simulink model "SMC_sim"  (R2024b)
settings: Solver=ode5  StartTime=0.0  StopTime=tf  FixedStep=dt  RelTol=1e-3
values from neighbouring files (symbols this model uses):
  A = double(subs(jacobian(x_dot, x_vars), [x_vars;u], [x_star; u_star]))    [inverted_pend_SMC.m]
  B = double(subs(jacobian(x_dot, u), [x_vars;u], [x_star; u_star]))    [inverted_pend_SMC.m]
  C = [1,0,0,0; 0,0,1,0]    [inverted_pend_SMC.m]
  eta = 100    [inverted_pend_SMC.m]
  L = place(A', C', poles_obsv)'    [inverted_pend_SMC.m]
  Phi = 0.1    [inverted_pend_SMC.m]
  r_pulley = 1.528*25.4/2000    (= 0.0194056)    [inverted_pend_SMC.m]
  x0 = [0; 0; -9*pi/180; 0]    [inverted_pend_SMC.m]
  x_star = [0;0;0;0]    [inverted_pend_SMC.m]
undefined symbols (not defined in the file or in its folder): K, params
libraries: simulink_extras x1
settings Model: Creator=johnc  LastModifiedBy=jcglenn

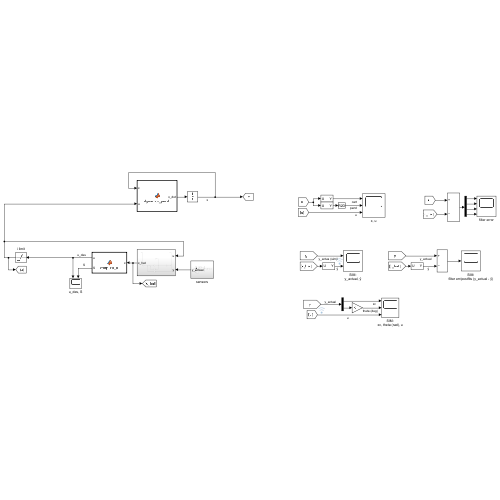
[thumbnail: Simulink's stored preview of the top-level diagram]
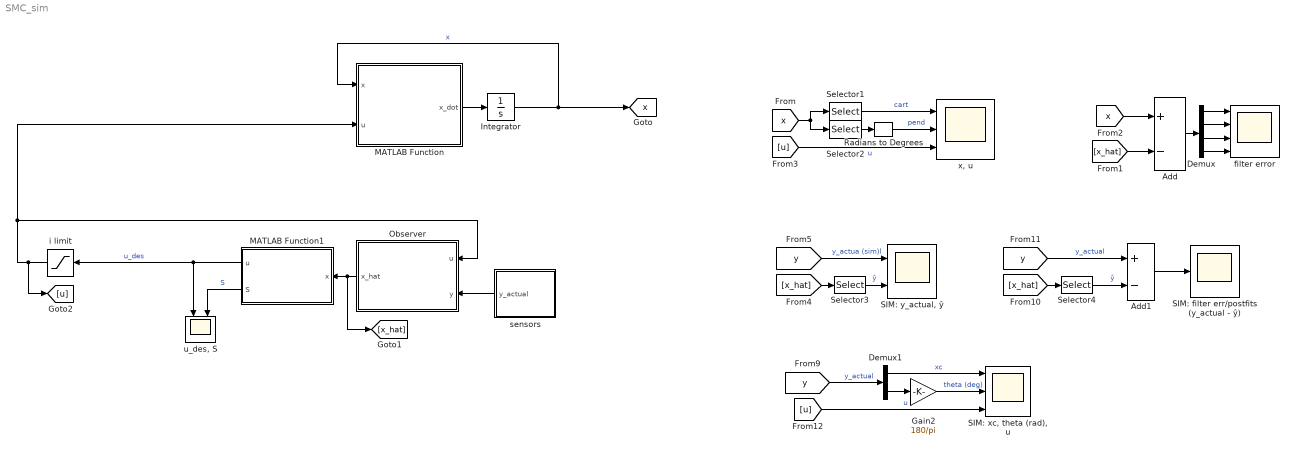
== system SMC_sim ==
  Add : Sum  Inputs=+-
  Add1 : Sum  Inputs=+-
  Demux : Demux
  Demux1 : Demux  Outputs=2
  Gain2 : Gain  Gain=180/pi
  Integrator : Integrator  InitialCondition=x0
  MATLAB Function : MATLAB Function  TreatAsAtomicUnit=on
  MATLAB Function1 : MATLAB Function  TreatAsAtomicUnit=on
  Observer : Subsystem
  Radians to Degrees : simulink_extras/Transformations/Radians to Degrees
  SIM: filter err/postfits (y_actual - ŷ) : Scope
  "SIM: xc, theta (rad), u" : Scope  NumInputPorts=3
  "SIM: y_actual, ŷ" : Scope  NumInputPorts=2
  Selector1 : Selector  InputPortWidth=4  IndexOptions=Index vector (dialog)  Indices=[1 2]  OutputSizes=1
  Selector2 : Selector  InputPortWidth=4  IndexOptions=Index vector (dialog)  Indices=[3 4]  OutputSizes=1
  Selector3 : Selector  InputPortWidth=4  IndexOptions=Index vector (dialog)  Indices=[1 3]  OutputSizes=1
  Selector4 : Selector  InputPortWidth=4  IndexOptions=Index vector (dialog)  Indices=[1 3]  OutputSizes=1
  filter error : Scope  NumInputPorts=4
  i limit : Saturate  UpperLimit=5.1  LowerLimit=-5.1
  sensors : Subsystem
  "u_des, S" : Scope  NumInputPorts=2
  "x, u" : Scope  NumInputPorts=3
  tag scope: x=global
  wires:
  MATLAB Function/1(x_dot) -> Integrator/1
  Integrator/1 -> [x], MATLAB Function/1(x)  "x"
  Observer/1(x_hat) -> MATLAB Function1/1(x), [x_hat]
  [x] -> Selector1/1, Selector2/1
  Selector1/1 -> "x, u"/1  "cart"
  Selector2/1 -> Radians to Degrees/1
  [x] -> Add/1
  [x_hat] -> Add/2
  Add/1 -> Demux/1
  Demux/1 -> filter error/1
  Demux/2 -> filter error/2
  Demux/3 -> filter error/3
  Demux/4 -> filter error/4
  [u] -> "x, u"/3  "u"
  MATLAB Function1/1(u) -> "u_des, S"/1, i limit/1  "u_des"
  i limit/1 -> [u], Observer/1(u), MATLAB Function/2(u)
  MATLAB Function1/2(S) -> "u_des, S"/2  "S"
  Radians to Degrees/1 -> "x, u"/2  "pend"
  sensors/1(y_actual) -> Observer/2(y)
  Selector4/1 -> Add1/2  "ŷ"
  [y] -> "SIM: y_actual, ŷ"/1  "y_actua (sim)l"
  Selector3/1 -> "SIM: y_actual, ŷ"/2  "ŷ"
  [x_hat] -> Selector4/1
  [y] -> Add1/1  "y_actual"
  [x_hat] -> Selector3/1
  Add1/1 -> SIM: filter err/postfits (y_actual - ŷ)/1
  Gain2/1 -> "SIM: xc, theta (rad), u"/2  "theta (deg)"
  Demux1/1 -> "SIM: xc, theta (rad), u"/1  "xc"
  [y] -> Demux1/1  "y_actual"
  Demux1/2 -> Gain2/1
  [u] -> "SIM: xc, theta (rad), u"/3  "u"

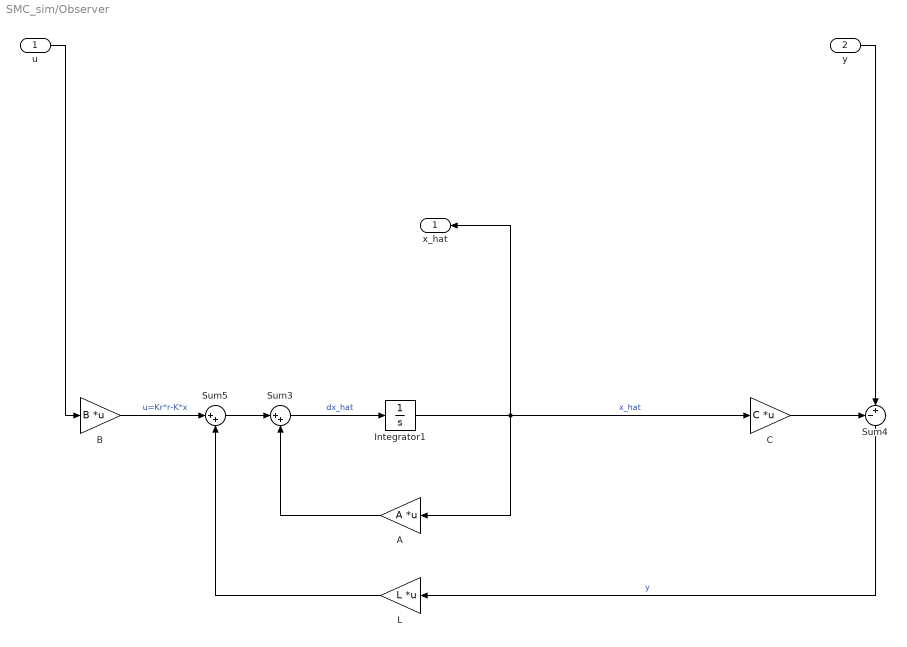
== system SMC_sim/Observer ==
  u : Inport
  y : Inport  Port=2
  A : Gain  Gain=A  Multiplication=Matrix(K*u)
  B : Gain  Gain=B  Multiplication=Matrix(K*u)
  C : Gain  Gain=C  Multiplication=Matrix(K*u)
  Integrator1 : Integrator  InitialCondition=x0-x_star
  L : Gain  Gain=L  Multiplication=Matrix(K*u)
  Sum3 : Sum  Inputs=|++
  Sum4 : Sum  Inputs=-+|
  Sum5 : Sum  Inputs=|++
  x_hat : Outport
  wires:
  C/1 -> Sum4/1
  Integrator1/1 -> x_hat/1, C/1, A/1  "x_hat"
  Sum5/1 -> Sum3/1
  L/1 -> Sum5/2
  A/1 -> Sum3/2
  Sum4/1 -> L/1  "y"
  Sum3/1 -> Integrator1/1  "dx_hat"
  B/1 -> Sum5/1  "u=Kr*r-K*x"
  u/1 -> B/1
  y/1 -> Sum4/2

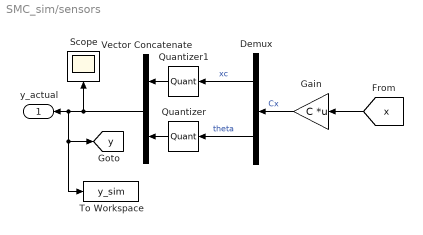
== system SMC_sim/sensors ==
  Demux : Demux  Outputs=2
  Gain : Gain  Gain=C  Multiplication=Matrix(K*u)
  Quantizer : Quantizer  QuantizationInterval=2*pi/10000
  Quantizer1 : Quantizer  QuantizationInterval=2*pi*r_pulley/10000
  Scope : Scope
  To Workspace : ToWorkspace  VariableName=y_sim  SampleTime=-1
  Vector Concatenate : Concatenate  Mode=Multidimensional array
  y_actual : Outport
  tag scope: y=global
  wires:
  Demux/1 -> Quantizer1/1  "xc"
  Demux/2 -> Quantizer/1  "theta"
  Quantizer1/1 -> Vector Concatenate/1
  Quantizer/1 -> Vector Concatenate/2
  [x] -> Gain/1
  Vector Concatenate/1 -> To Workspace/1, [y], y_actual/1, Scope/1
  Gain/1 -> Demux/1  "Cx"

== matlab function SMC_sim/MATLAB Function1 ==
  data: x input; K parameter; Phi parameter; eta parameter; u output; params parameter; S output
function [u, S] = compute_u(x, K, Phi, eta, params)

g = params.g;
mc = params.mc;
mp = params.mp;
Jp = params.Jp;
bc = params.bc;
bp = params.bp;
Lp = params.Lp;
r_pulley = params.r_pulley;
Ke = params.Ke;

x1 = x(1);
x2 = x(2);
x3 = x(3);
x4 = x(4);

F = [x2;
     -(bc*x2 + Lp*mp*x4^2*sin(x3) + (Lp*mp*cos(x3)*(bp*x4 - Lp*g*mp*sin(x3)))/(mp*Lp^2 + Jp))/(mc + mp - (Lp^2*mp^2*cos(x3)^2)/(mp*Lp^2 + Jp));
     x4;
     -(bp*x4 - Lp*g*mp*sin(x3) + (Lp*mp*cos(x3)*(Lp*mp*sin(x3)*x4^2 + bc*x2))/(mc + mp))/(Jp + Lp^2*mp - (Lp^2*mp^2*cos(x3)^2)/(mc + mp))];

G = [0;
     Ke/(r_pulley*(mc + mp - (Lp^2*mp^2*cos(x3)^2)/(mp*Lp^2 + Jp)));
     0;
     (Ke*Lp*mp*cos(x3))/(r_pulley*(mc + mp)*(Jp + Lp^2*mp - (Lp^2*mp^2*cos(x3)^2)/(mc + mp)))];

S = K*x(:);

h = -eta*min(1, max(-1, S/Phi));

% u = (K*G)\(h - K*F);

u_1 = -(K*G)\(K*F);
u_2 = (K*G)\h;
u = u_1 + u_2;

== matlab function SMC_sim/MATLAB Function ==
  data: x input; x_dot output; u input; params parameter
function x_dot  = dynamics_pend(x, u, params)

g = params.g;
mc = params.mc;
mp = params.mp;
Jp = params.Jp;
bc = params.bc;
bp = params.bp;
Lp = params.Lp;
r_pulley = params.r_pulley;
Ke = params.Ke;
Fc = params.Fc;

x1 = x(1);
x2 = x(2);
x3 = x(3);
x4 = x(4);

F_fric = Fc*tanh(100*x2);
% F_fric = 0; %COMMENT OUT

x1_dot = x2;
x2_dot = (Ke*u/r_pulley - bc*x2 - F_fric - mp*Lp*x4^2*sin(x3) + mp*Lp*cos(x3)*(-bp*x4 + mp*g*Lp*sin(x3))/(mp*Lp^2 + Jp))*1/(mc + mp - mp^2*Lp^2*cos(x3)^2/(mp*Lp^2 + Jp));
x3_dot = x4;
x4_dot = (-bp*x4 + mp*g*Lp*sin(x3) + mp*Lp*cos(x3)*(Ke*u/r_pulley - bc*x2 - mp*Lp*x4^2*sin(x3))/(mc + mp))*1/(mp*Lp^2 + Jp - mp^2*Lp^2*cos(x3)^2/(mc + mp));

x_dot = [x1_dot; x2_dot; x3_dot; x4_dot];
